simulink model "aircraft_model"  (R2014b)
settings: Solver=ode45  StartTime=0.0  StopTime=10.0  FixedStep=0.001  RelTol=1e-3
values from neighbouring files (symbols this model uses):
  h0 = 1.5    [sim_data.mat]    (also in simulation_framework.m)
  m_p = 0.64    [sim_data.mat]    (also in simulation_framework.m)
  m_phi = 1.21846967915e-05    [sim_data.mat]    (also in simulation_framework.m)
  m_v = 0.25    [sim_data.mat]    (also in simulation_framework.m)
  m_v_air = 0.01    [sim_data.mat]    (also in simulation_framework.m)
  p0 = [2 2]    [sim_data.mat]    (also in simulation_framework.m = [2;2])
  phi_max = 0.523598775598    [sim_data.mat]    (also in simulation_framework.m)
  q = q+q_add    [high_level.m]    (also in start_script.m = 0.005)
  r = d+db/norm(db)*ddr    [lateral_guidance.m]
  seed_p_pdot = [814724 905792 12707 913377 6692 975494]    [sim_data.mat]    (also in simulation_framework.m = [10;2;0.01;2311;132;453287])
  seed_phi = 54689    [sim_data.mat]    (also in simulation_framework.m = 20143)
  seed_v_air = 27849822    [sim_data.mat]    (also in simulation_framework.m = 33)
  Tctrl = 0.1    [sim_data.mat]    (also in simulation_framework.m)
  Ts = 0.1    [sim_data.mat]    (also in simulation_framework.m)
  Ts_p_pdot = 2    [sim_data.mat]    (also in simulation_framework.m)
  Ts_phi = 1    [sim_data.mat]    (also in simulation_framework.m)
  Ts_v_air = 1    [sim_data.mat]    (also in simulation_framework.m)
  VTd = 10    [sim_data.mat]    (also in simulation_framework.m)
  Vw = norm(w)    [findxi.m]    (also in sim_data.mat = 2; simulation_framework.m = 1)
  xi0 = 1.57079632679    [sim_data.mat]    (also in simulation_framework.m = double(findxi(xig0,VTd,w)))
  xiw = atan2(w(2),w(1))    [findxi.m]    (also in sim_data.mat = 4.71238898038; simulation_framework.m = 4.71238898038)
undefined symbols (not defined in the file or in its folder): F, Light, MIL, sigbuilder_block
libraries: aerolibwind2 x2, aerolibtransform2 x1, simulink x1
settings Model: Creator=tstastny  LastModifiedBy=Maverick
settings SolverCC: ZeroCrossAlgorithm=Adaptive
settings OptimizationCC: UseDivisionForNetSlopeComputation=off  SimCompilerOptimization=off
settings DebuggingCC: FrameProcessingCompatibilityMsg=error
settings RTWCC: RTWCompilerOptimization=off

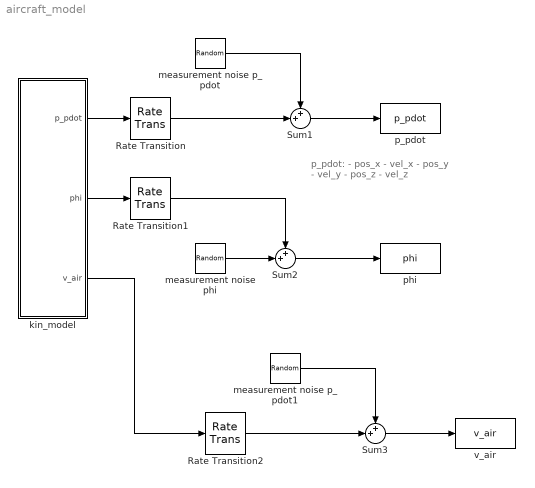
== system aircraft_model ==
  note: p_pdot:  - pos_x
      |               - vel_x
      |               - pos_y
      |               - vel_y
      |               - pos_z
      |               - vel_z
  Rate Transition : RateTransition  Integrity=off  OutPortSampleTime=Ts_p_pdot
  Rate Transition1 : RateTransition  Integrity=off  OutPortSampleTime=Ts_phi
  Rate Transition2 : RateTransition  Integrity=off  OutPortSampleTime=Ts_v_air
  Sum1 : Sum  Inputs=++|  SampleTime=Ts_p_pdot
  Sum2 : Sum  Inputs=++|  SampleTime=Ts_phi
  Sum3 : Sum  Inputs=++|  SampleTime=Ts_v_air
  kin_model : Subsystem
  measurement noise p_pdot : RandomNumber  Variance=[m_p;m_v;m_p;m_v;m_p;m_v]  Seed=seed_p_pdot  SampleTime=Ts_p_pdot
  measurement noise p_pdot1 : RandomNumber  Variance=[m_v_air]  Seed=seed_v_air  SampleTime=Ts_v_air
  measurement noise phi : RandomNumber  Variance=m_phi  Seed=seed_phi  SampleTime=Ts_phi
  p_pdot : ToWorkspace  VariableName=p_pdot  SaveFormat=Structure With Time  SampleTime=-1
  phi : ToWorkspace  VariableName=phi  SaveFormat=Structure With Time  SampleTime=-1
  v_air : ToWorkspace  VariableName=v_air  SaveFormat=Structure With Time  SampleTime=-1
  wires:
  measurement noise p_pdot/1 -> Sum1/1
  measurement noise phi/1 -> Sum2/2
  kin_model/2(phi) -> Rate Transition1/1
  kin_model/1(p_pdot) -> Rate Transition/1
  Rate Transition/1 -> Sum1/2
  Sum1/1 -> p_pdot/1
  Rate Transition1/1 -> Sum2/1
  Sum2/1 -> phi/1
  measurement noise p_pdot1/1 -> Sum3/1
  Rate Transition2/1 -> Sum3/2
  Sum3/1 -> v_air/1
  kin_model/3(v_air) -> Rate Transition2/1

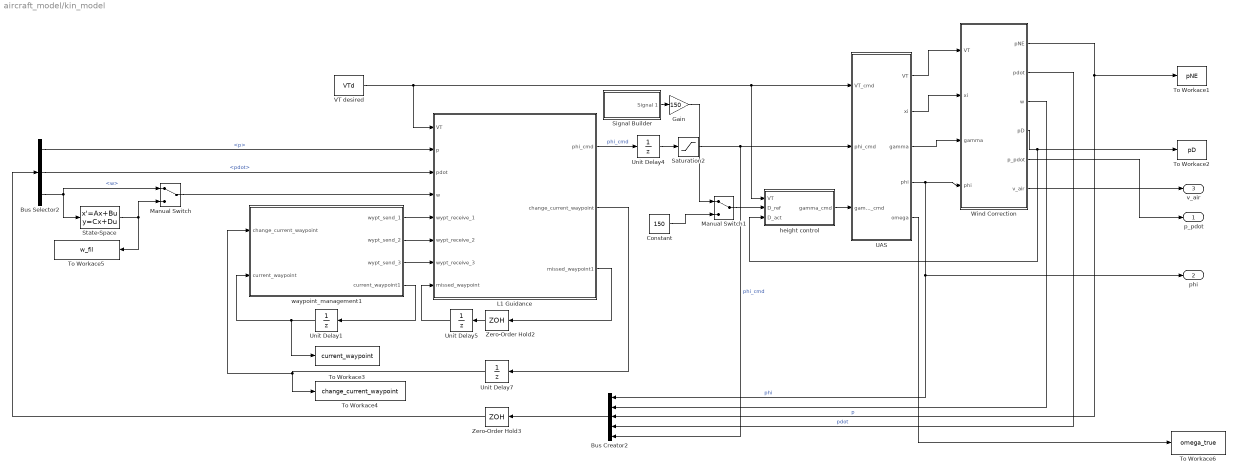
== system aircraft_model/kin_model ==
  Bus Creator2 : BusCreator  Inputs=5
  Bus Selector2 : BusSelector  OutputSignals=p,pdot,w
  Constant : Constant  Value=150  SampleTime=Ts
  Gain : Gain  Gain=150
  L1 Guidance : MATLAB Function  TreatAsAtomicUnit=on  SystemSampleTime=Tctrl
  Manual Switch : ManualSwitch
  Manual Switch1 : ManualSwitch
  Saturation2 : Saturate  UpperLimit=phi_max  LowerLimit=-phi_max
  Signal Builder : Subsystem  Tag=STV Subsys  LoadFcn=sigbuilder_block('load',[0 51 1440 753 ]);  StartFcn=sigbuilder_block('start');  StopFcn=sigbuilder_block('stop');  ClipboardFcn=sigbuilder_block('clipboard');  mask(Sigbuilder block){}
      mask help: Simulink:masks:SigbuilderBlock_MD
      mask init:
      | if ~strcmp(get_param(bdroot(gcbh),'SimulationStatus'),'stopped') tuvar = sigbuilder_block('maskInit'); end
      settings: CopyFcn=sigbuilder_block('copy');  DeleteFcn=sigbuilder_block('delete');  ModelCloseFcn=sigbuilder_block('modelClose');  PreSaveFcn=sigbuilder_block('preSave');  PauseFcn=sigbuilder_block('pause');  ContinueFcn=sigbuilder_block('continue');  NameChangeFcn=sigbuilder_block('namechange');  OpenFcn=sigbuilder_block('open',[437.6 199.2 550.4 400 ]);  CloseFcn=sigbuilder_block('close');
      mask Display: plot(0, 0, 100, 100,[2, 2, 32, 32, 2], [68, 8, 8, 68, 68],[32, 2], [38, 38], [32, 19, 2],[53, 60, 44], [32, 17, 17, 2],[16, 16, 31, 31]);txt = getActiveGroup(gcbh);text(2, 100, txt,'verticalAlignment', 'top');
  State-Space : StateSpace  A=-1*eye(2)  B=1*eye(2)  C=eye(2)  D=zeros(2)  X0=double([Vw*cos(xiw);Vw*sin(xiw)])
  To Workace1 : ToWorkspace  VariableName=pNE  SaveFormat=Structure With Time  SampleTime=Ts
  To Workace2 : ToWorkspace  VariableName=pD  SaveFormat=Structure With Time  SampleTime=Ts
  To Workace3 : ToWorkspace  VariableName=current_waypoint  SaveFormat=Structure With Time  SampleTime=Ts
  To Workace4 : ToWorkspace  VariableName=change_current_waypoint  SaveFormat=Structure With Time  SampleTime=Ts
  To Workace5 : ToWorkspace  VariableName=w_fil  SaveFormat=Structure With Time  SampleTime=Ts
  To Workace6 : ToWorkspace  VariableName=omega_true  SaveFormat=Structure With Time  SampleTime=Ts
  "UAS " : Subsystem
  Unit Delay1 : UnitDelay  InitialCondition=1  SampleTime=0.001
  Unit Delay4 : UnitDelay  SampleTime=0.001
  Unit Delay5 : UnitDelay  SampleTime=0.001
  Unit Delay7 : UnitDelay  SampleTime=0.001
  VT desired : Constant  Value=VTd
  Wind Correction : Subsystem
  Zero-Order Hold2 : ZeroOrderHold  SampleTime=0.001
  Zero-Order Hold3 : ZeroOrderHold  SampleTime=Tctrl
  height control : Subsystem
  waypoint_management1 : MATLAB Function  TreatAsAtomicUnit=on  SystemSampleTime=Tctrl
  p_pdot : Outport
  phi : Outport  Port=2
  v_air : Outport  Port=3
  wires:
  "UAS "/1(VT) -> Wind Correction/1(VT)
  "UAS "/2(xi) -> Wind Correction/2(xi)
  "UAS "/4(phi) -> phi/1, Bus Creator2/1, Wind Correction/4(phi)  "phi"
  Wind Correction/1(pNE) -> Bus Creator2/3, To Workace1/1  "p"
  Wind Correction/2(pdot) -> Bus Creator2/4  "pdot"
  Bus Creator2/1 -> Zero-Order Hold3/1
  Zero-Order Hold3/1 -> Bus Selector2/1
  Bus Selector2/1 -> L1 Guidance/2(p)  "<p>"
  Bus Selector2/2 -> L1 Guidance/3(pdot)  "<pdot>"
  Saturation2/1 -> "UAS "/2(phi_cmd), Bus Creator2/5  "phi_cmd"
  waypoint_management1/4(current_waypoint1) -> Unit Delay1/1
  Unit Delay1/1 -> To Workace3/1, waypoint_management1/2(current_waypoint)
  L1 Guidance/2(change_current_waypoint) -> Unit Delay7/1
  waypoint_management1/3(wypt_send_3) -> L1 Guidance/7(wypt_receive_3)
  waypoint_management1/2(wypt_send_2) -> L1 Guidance/6(wypt_receive_2)
  waypoint_management1/1(wypt_send_1) -> L1 Guidance/5(wypt_receive_1)
  L1 Guidance/3(missed_waypoint1) -> Zero-Order Hold2/1
  Zero-Order Hold2/1 -> Unit Delay5/1
  Wind Correction/3(w) -> Bus Creator2/2
  Bus Selector2/3 -> State-Space/1, Manual Switch/1  "<w>"
  State-Space/1 -> To Workace5/1, Manual Switch/2
  Manual Switch/1 -> L1 Guidance/4(w)
  Unit Delay4/1 -> Saturation2/1
  Unit Delay5/1 -> L1 Guidance/8(missed_waypoint)
  Unit Delay7/1 -> To Workace4/1, waypoint_management1/1(change_current_waypoint)
  L1 Guidance/1(phi_cmd) -> Unit Delay4/1  "phi_cmd"
  Wind Correction/4(pD) -> height control/3(D_act), To Workace2/1
  "UAS "/3(gamma) -> Wind Correction/3(gamma)
  height control/1(gamma_cmd) -> "UAS "/3(gamma_cmd)
  VT desired/1 -> L1 Guidance/1(VT), "UAS "/1(VT_cmd), height control/1(VT)
  Wind Correction/5(p_pdot) -> p_pdot/1
  "UAS "/5(omega) -> To Workace6/1
  Constant/1 -> Manual Switch1/2
  Manual Switch1/1 -> height control/2(D_ref)
  Wind Correction/6(v_air) -> v_air/1
  Gain/1 -> Manual Switch1/1
  Signal Builder/1(Signal 1) -> Gain/1

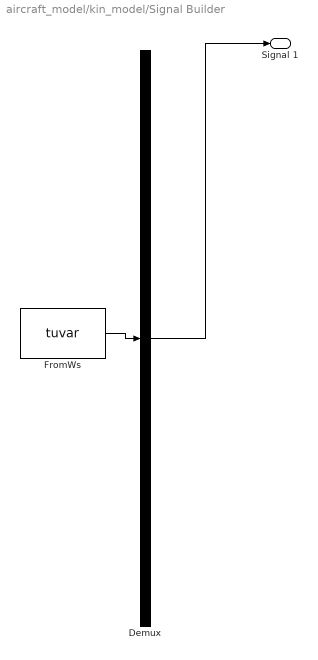
== system aircraft_model/kin_model/Signal Builder ==
  Demux : Demux  Tag=STV Demux  Outputs=1
  FromWs : FromWorkspace  Tag=STV FromWs  VariableName=tuvar  SampleTime=0
      SigBuilderData=|
      | common.afterFinalStr = 'Extrapolate'
      | common.sampleTime = 0
      | dataSet.timeRange = [0 180]
      | dataSet.name = 'Group 1'
      | sbobj.Groups.Name = 'Group 1'
      | sbobj.Groups.Signals.Name = 'Signal 1'
      | sbobj.Groups.Signals.XData = [0 2 10 15 17 20 25 40 60 80 90 100 140 180]
      | sbobj.Groups.Signals.YData = [0 0.008 0.02 0.044 0.052 0.066 0.094 0.192 0.296 0.362 0.362 0.324 0.184 0.048]
      | sbobj.Groups.TimeRange = [0 180]
  Signal 1 : Outport  Tag=STV Outport
  wires:
  Demux/1 -> Signal 1/1
  FromWs/1 -> Demux/1

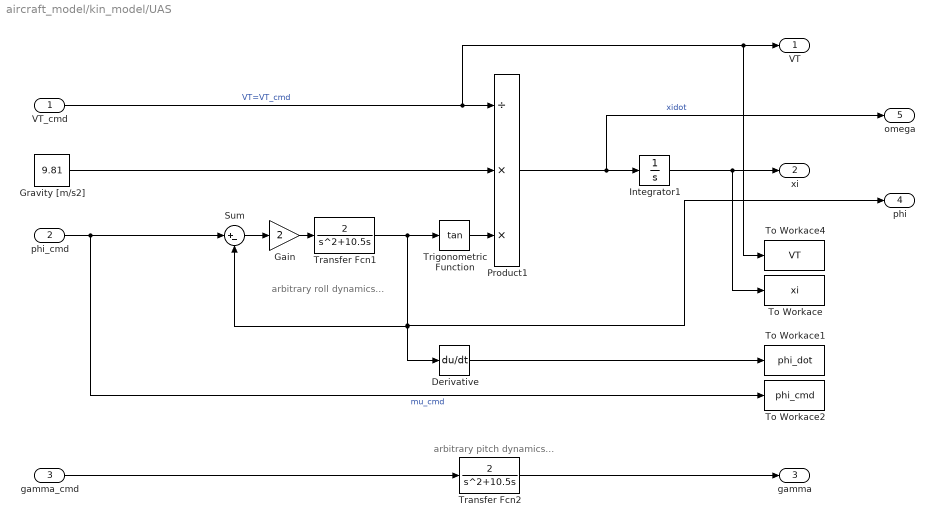
== system aircraft_model/kin_model/UAS  ==
  note: arbitrary roll dynamics...
  note: arbitrary pitch dynamics...
  VT_cmd : Inport
  phi_cmd : Inport  Port=2
  gamma_cmd : Inport  Port=3
  Derivative : Derivative
  Gain : Gain  Gain=2
  Gravity [m/s2] : Constant  Value=9.81
  Integrator1 : Integrator  InitialCondition=xi0
  Product1 : Product  Inputs=/**
  Sum : Sum  Inputs=|+-
  To Workace : ToWorkspace  VariableName=xi  SaveFormat=Structure With Time  SampleTime=Ts
  To Workace1 : ToWorkspace  VariableName=phi_dot  SaveFormat=Structure With Time  SampleTime=Ts
  To Workace2 : ToWorkspace  VariableName=phi_cmd  SaveFormat=Structure With Time  SampleTime=Ts
  To Workace4 : ToWorkspace  VariableName=VT  SaveFormat=Structure With Time  SampleTime=Ts
  Transfer Fcn1 : TransferFcn  Numerator=[2]  Denominator=[1 10.5 0]
  Transfer Fcn2 : TransferFcn  Numerator=[2]  Denominator=[1 10.5 0]
  Trigonometric Function : Trigonometry  Operator=tan
  VT : Outport
  xi : Outport  Port=2
  gamma : Outport  Port=3
  phi : Outport  Port=4
  omega : Outport  Port=5
  wires:
  phi_cmd/1 -> Sum/1, To Workace2/1  "mu_cmd"
  Trigonometric Function/1 -> Product1/3
  Gravity [m/s2]/1 -> Product1/2
  VT_cmd/1 -> To Workace4/1, VT/1, Product1/1  "VT=VT_cmd"
  Product1/1 -> omega/1, Integrator1/1  "xidot"
  Transfer Fcn1/1 -> Derivative/1, Sum/2, phi/1, Trigonometric Function/1
  Derivative/1 -> To Workace1/1
  Gain/1 -> Transfer Fcn1/1
  Sum/1 -> Gain/1
  Integrator1/1 -> To Workace/1, xi/1
  gamma_cmd/1 -> Transfer Fcn2/1
  Transfer Fcn2/1 -> gamma/1

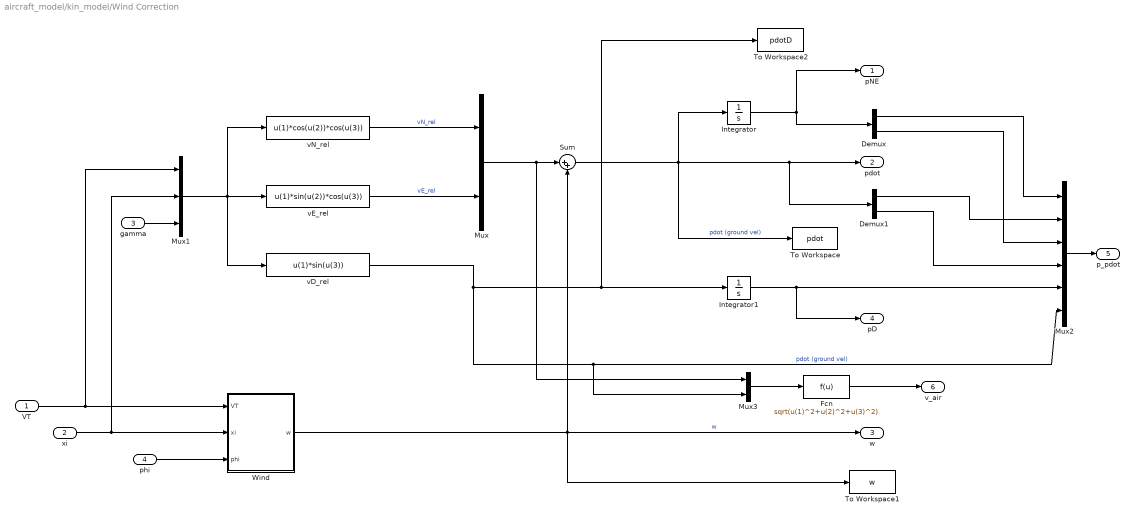
== system aircraft_model/kin_model/Wind Correction ==
  VT : Inport
  xi : Inport  Port=2
  gamma : Inport  Port=3
  phi : Inport  Port=4
  Demux : Demux  Outputs=2
  Demux1 : Demux  Outputs=2
  Fcn : Fcn  Expr=sqrt(u(1)^2+u(2)^2+u(3)^2)
  Integrator : Integrator  InitialCondition=p0
  Integrator1 : Integrator  InitialCondition=h0
  Mux : Mux  Inputs=2
  Mux1 : Mux  Inputs=3
  Mux2 : Mux  Inputs=6
  Mux3 : Mux  Inputs=2
  Sum : Sum  Inputs=|++
  To Workspace : ToWorkspace  VariableName=pdot  SaveFormat=Structure With Time  SampleTime=Ts
  To Workspace1 : ToWorkspace  VariableName=w  SaveFormat=Structure With Time  SampleTime=Ts
  To Workspace2 : ToWorkspace  VariableName=pdotD  SaveFormat=Structure With Time  SampleTime=Ts
  Wind : Subsystem
  vD_rel : Fcn  Expr=u(1)*sin(u(3))  SampleTime=Ts
  vE_rel : Fcn  Expr=u(1)*sin(u(2))*cos(u(3))  SampleTime=Ts
  vN_rel : Fcn  Expr=u(1)*cos(u(2))*cos(u(3))  SampleTime=Ts
  pNE : Outport  PortDimensions=2
  pdot : Outport  Port=2  PortDimensions=2
  w : Outport  Port=3  PortDimensions=2
  pD : Outport  Port=4
  p_pdot : Outport  Port=5
  v_air : Outport  Port=6
  wires:
  VT/1 -> Mux1/1, Wind/1(VT)
  Wind/1(w) -> To Workspace1/1, Sum/2, w/1  "w"
  xi/1 -> Mux1/2, Wind/2(xi)
  phi/1 -> Wind/3(phi)
  Mux/1 -> Mux3/1, Sum/1
  Sum/1 -> Integrator/1, Demux1/1, pdot/1, To Workspace/1  "pdot (ground vel)"
  Integrator/1 -> Demux/1, pNE/1
  gamma/1 -> Mux1/3
  vN_rel/1 -> Mux/1  "vN_rel"
  vE_rel/1 -> Mux/2  "vE_rel"
  Mux1/1 -> vN_rel/1, vD_rel/1, vE_rel/1
  Integrator1/1 -> pD/1, Mux2/5
  vD_rel/1 -> Mux3/2, Mux2/6, To Workspace2/1, Integrator1/1  "pdot (ground vel)"
  Mux2/1 -> p_pdot/1
  Demux/1 -> Mux2/1
  Demux/2 -> Mux2/3
  Demux1/2 -> Mux2/4
  Demux1/1 -> Mux2/2
  Fcn/1 -> v_air/1
  Mux3/1 -> Fcn/1

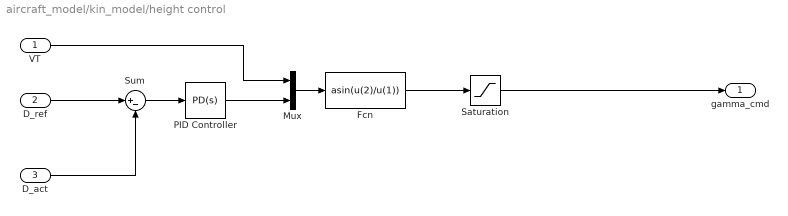
== system aircraft_model/kin_model/height control ==
  VT : Inport
  D_ref : Inport  Port=2
  D_act : Inport  Port=3
  Fcn : Fcn  Expr=asin(u(2)/u(1))  SampleTime=Ts
  Mux : Mux  Inputs=2
  PID Controller : simulink/Continuous/PID Controller  Controller=PD  TimeDomain=Continuous-time  SampleTime=-1  IntegratorMethod=Forward Euler  FilterMethod=Forward Euler  Form=Parallel  P=5  I=1  D=10  N=100  InitialConditionSource=internal  InitialConditionForIntegrator=0  InitialConditionForFilter=0  ExternalReset=none  LimitOutput=off  UpperSaturationLimit=inf  LowerSaturationLimit=-inf  LinearizeAsGain=on  AntiWindupMode=none  Kb=1  TrackingMode=off  Kt=1  PParamMin=[]  PParamMax=[]  IParamMin=[]  IParamMax=[]  DParamMin=[]  DParamMax=[]  NParamMin=[]  NParamMax=[]  KbParamMin=[]  KbParamMax=[]  KtParamMin=[]  KtParamMax=[]  POutMin=[]  POutMax=[]  IOutMin=[]  IOutMax=[]  DOutMin=[]  DOutMax=[]  NOutMin=[]  NOutMax=[]  KbOutMin=[]  KbOutMax=[]  KtOutMin=[]  KtOutMax=[]  IntegratorOutMin=[]  IntegratorOutMax=[]  FilterOutMin=[]  FilterOutMax=[]  SumOutMin=[]  SumOutMax=[]  SumI1OutMin=[]  SumI1OutMax=[]  SumI2OutMin=[]  SumI2OutMax=[]  SumI3OutMin=[]  SumI3OutMax=[]  SumDOutMin=[]  SumDOutMax=[]  SaturationOutMin=[]  SaturationOutMax=[]  IntegratorContinuousStateAttributes=''  IntegratorStateMustResolveToSignalObject=off  IntegratorRTWStateStorageClass=Auto  FilterContinuousStateAttributes=''  FilterStateMustResolveToSignalObject=off  FilterRTWStateStorageClass=Auto  DifferentiatorICPrevScaledInput=0  DifferentiatorOutMin=[]  DifferentiatorOutMax=[]  UseFilter=on
  Saturation : Saturate  UpperLimit=phi_max  LowerLimit=-phi_max
  Sum : Sum  Inputs=|+-
  gamma_cmd : Outport
  wires:
  D_ref/1 -> Sum/1
  Fcn/1 -> Saturation/1
  PID Controller/1 -> Mux/2
  D_act/1 -> Sum/2
  Sum/1 -> PID Controller/1
  VT/1 -> Mux/1
  Mux/1 -> Fcn/1
  Saturation/1 -> gamma_cmd/1

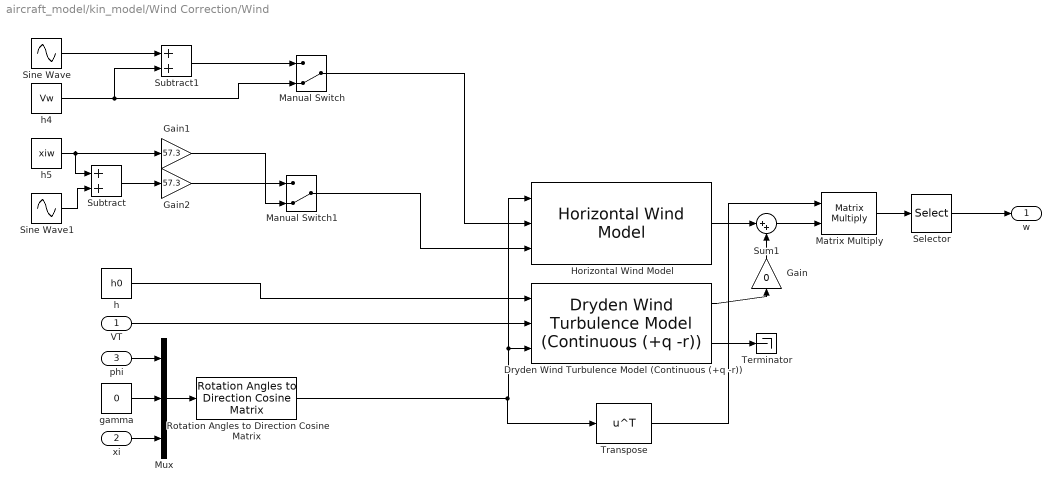
== system aircraft_model/kin_model/Wind Correction/Wind ==
  VT : Inport
  xi : Inport  Port=2
  phi : Inport  Port=3
  Dryden Wind Turbulence Model (Continuous (+q -r)) : aerolibwind2/Dryden Wind Turbulence Model  (Continuous (+q -r))  units=Metric (MKS)  spec=MIL-F-8785C  model=Continuous Dryden (+q -r)  W20=Vw  Wdeg=xiw  TurbProb=10^-2 - Light  L_high=533.4  Wingspan=b_uas  ts=0.01  Seed=[23341 23342 23343 23344]  T_on=on
  Gain : Gain  Gain=0
  Gain1 : Gain  Gain=57.3
  Gain2 : Gain  Gain=57.3
  Horizontal Wind Model : aerolibwind2/Horizontal Wind Model  units=Metric (MKS)  Vw_source=External  Vwind=Vw  W_source=External  Wdeg=xiw
  Manual Switch : ManualSwitch  CurrentSetting=0
  Manual Switch1 : ManualSwitch  CurrentSetting=0
  Matrix Multiply : Product  Multiplication=Matrix(*)
  Mux : Mux  Inputs=3
  Rotation Angles to Direction Cosine Matrix : aerolibtransform2/Rotation Angles to Direction Cosine Matrix  rotationOrder=ZYX
  Selector : Selector  InputPortWidth=3  Indices=[1 2]
  Sine Wave : Sin  Amplitude=3  Bias=-1  Frequency=0.05  SampleTime=0
  Sine Wave1 : Sin  Amplitude=30*pi/180  Frequency=0.1  Phase=35*pi/180  SampleTime=0
  Subtract : Sum
  Subtract1 : Sum
  Sum1 : Sum  Inputs=|++
  Terminator : Terminator
  Transpose : Math  Operator=transpose  SaturateOnIntegerOverflow=on
  gamma : Constant  Value=0
  h : Constant  Value=h0
  h4 : Constant  Value=Vw
  h5 : Constant  Value=xiw
  w : Outport
  wires:
  Dryden Wind Turbulence Model (Continuous (+q -r))/2 -> Terminator/1
  Mux/1 -> Rotation Angles to Direction Cosine Matrix/1
  Rotation Angles to Direction Cosine Matrix/1 -> Transpose/1, Dryden Wind Turbulence Model (Continuous (+q -r))/3, Horizontal Wind Model/1
  h/1 -> Dryden Wind Turbulence Model (Continuous (+q -r))/1
  VT/1 -> Dryden Wind Turbulence Model (Continuous (+q -r))/2
  Horizontal Wind Model/1 -> Sum1/1
  Dryden Wind Turbulence Model (Continuous (+q -r))/1 -> Gain/1
  Transpose/1 -> Matrix Multiply/1
  Sum1/1 -> Matrix Multiply/2
  Selector/1 -> w/1
  Matrix Multiply/1 -> Selector/1
  xi/1 -> Mux/3
  gamma/1 -> Mux/2
  phi/1 -> Mux/1
  Gain/1 -> Sum1/2
  h4/1 -> Manual Switch/2, Subtract1/2
  Sine Wave/1 -> Subtract1/1
  Subtract/1 -> Gain2/1
  h5/1 -> Subtract/1, Gain1/1
  Sine Wave1/1 -> Subtract/2
  Manual Switch1/1 -> Horizontal Wind Model/3
  Manual Switch/1 -> Horizontal Wind Model/2
  Subtract1/1 -> Manual Switch/1
  Gain2/1 -> Manual Switch1/1
  Gain1/1 -> Manual Switch1/2

== matlab function aircraft_model/kin_model/L1 Guidance ==
  data: VT input; p input size=2; pdot input size=2; w input size=2; wypt_receive_1 input Bus: wypt_send_1 size=1; phi_cmd output size=1; wypt_receive_2 input Bus: wypt_send_2 size=1; wypt_receive_3 input Bus: wypt_send_3 size=1; change_current_waypoint output size=1; missed_waypoint input size=1; missed_waypoint1 output size=1
function [phi_cmd,change_current_waypoint,missed_waypoint1] = L1Guidance(VT,p,pdot,w,wypt_receive_1,wypt_receive_2,wypt_receive_3,missed_waypoint)
%#codegen

wypts = [wypt_receive_1,wypt_receive_2,wypt_receive_3];

Rdefault = 70;
sdefault = 1;
change_current_waypoint = 0;
phi_cmd = 0;

% Wind speed estimate greater than airspeed
if norm(w) > 0.99*VT
    
    phi_cmd = 0;%over_airspeed(pdot,w,mumax);
    
elseif ~wypts(1).active && ~wypts(3).active % Only one active waypoint
    
%     [phi_cmd,LAflag] = ...
%         loiter(phi_cmd0,p,pdot,VT,w,g,wypts(2),mumax,loit_opt,LAgain,Lparams);

    phi_cmd = 0;

elseif wypts(2).wtype==1 % Loiter (unlimited, unless MAVLink says otherwise)
    
%     [phi_cmd,LAflag] = ...
%         loiter(phi_cmd0,p,pdot,VT,w,g,wypts(2),mumax,loit_opt,LAgain,Lparams);
    
elseif wypts(2).wtype==0 % Segment tracking
    
    if ~wypts(1).active || missed_waypoint % Inactive wypts 1 or missed wypts 2
        
        if norm(wypts(2).p-p)<wypts(2).param1
            
            if ~wypts(3).active % Terminal loiter
                
%                 [phi_cmd,LAflag] = ...
%                     loiter(phi_cmd0,p,pdot,VT,w,g,wypts(2),mumax,loit_opt,LAgain,Lparams);
                phi_cmd = 0;
                
            else % switch to next wypts pair
                
                a = wypts(2).p;
                b = wypts(3).p;
                phi_cmd = lateral_guidance(p,pdot,a,b);
                
            end
        
            missed_waypoint=0;
            change_current_waypoint=1;
            
        else % L1 guide from p to b
            
            a = p;
            b = wypts(2).p;
            phi_cmd = lateral_guidance(p,pdot,a,b);
        
        end
        
    elseif ~wypts(3).active % Terminal
        
        % check for missed..
        xi_track = atan2(wypts(2).p(2)-wypts(1).p(2),...
            wypts(2).p(2)-wypts(1).p(2));
        HINt = [cos(xi_track) sin(xi_track)];
        if HINt*(p-wypts(1).p) > HINt*(wypts(2).p-wypts(1).p)+wypts(2).param1
            missed_waypoint=1;
        end
        
        if norm(wypts(2).p-p)<wypts(2).param1
        % for now just keep going back to the same... should loiter
            
        	a = p;
            b = wypts(2).p;
            phi_cmd = lateral_guidance(p,pdot,a,b);
            
            change_current_waypoint=1;
            
        elseif missed_waypoint
            
        	a = p;
            b = wypts(2).p;
            phi_cmd = lateral_guidance(p,pdot,a,b);
        
        else
            
            a = wypts(1).p;
            b = wypts(2).p;
            phi_cmd = lateral_guidance(p,pdot,a,b);
        
        end
        
    else
        
        % check for missed..
        xi_track = atan2(wypts(2).p(2)-wypts(1).p(2),...
            wypts(2).p(2)-wypts(1).p(2));
        HINt = [cos(xi_track) sin(xi_track)];
        if HINt*(p-wypts(1).p) > HINt*(wypts(2).p-wypts(1).p)+wypts(2).param1
            missed_waypoint=1;
        end
        
        if norm(wypts(2).p-p)<wypts(2).param1 
            
            a = wypts(2).p;
            b = wypts(3).p;
            phi_cmd = lateral_guidance(p,pdot,a,b);
            
            change_current_waypoint=1;
        
        elseif missed_waypoint
            
            a = p;
            b = wypts(2).p;
            phi_cmd = lateral_guidance(p,pdot,a,b);
            
        else
            
            a = wypts(1).p;
            b = wypts(2).p;
            phi_cmd = lateral_guidance(p,pdot,a,b);
            
        end
             
    end

else % Level aircraft
    
    phi_cmd = 0;
    
end

missed_waypoint1 = missed_waypoint;

== matlab function aircraft_model/kin_model/waypoint_management1 ==
  data: wypts0 parameter size=sizewypts00; change_current_waypoint input size=1; wypt_send_1 output Bus: wypt_send_1 size=1; wypt_send_2 output Bus: wypt_send_2 size=1; wypt_send_3 output Bus: wypt_send_3 size=1; current_waypoint input size=1; current_waypoint1 output size=1
function [wypt_send_1,wypt_send_2,wypt_send_3,current_waypoint1] = ...
    waypoint_management(wypts0,change_current_waypoint,current_waypoint)
%#codegen
% ========================================================================

% This block is intended to mimic Mavlink waypoint switching logic

% ========================================================================

% - - - - - - -
% Waypoint info
% - - - - - - - 

% Empty waypoint
wyptsi = struct('active',0,...
                'wtype',0,...
                'p',zeros(2,1),...
                'param1',30,...
                'param2',0);

% Size of waypoint list
size_waypoint_list = size(wypts0,1);

% - - - - - - - - - - - - - - -
% Determine waypoint send list
% - - - - - - - - - - - - - - -

% Check for change
if change_current_waypoint
    
    % Reached end of list, loop back
    if current_waypoint == size_waypoint_list || size_waypoint_list == 1
        
        current_waypoint = 1;
        
    else
        
        current_waypoint = current_waypoint + 1;
        
    end
    
end

% - - - - - - - - -
% Waypoint send set
% - - - - - - - - - 

if size_waypoint_list == 1
    
    wypt_send_1 = wyptsi;
    wypt_send_2 = wypts0;
    wypt_send_3 = wyptsi;
    
elseif size_waypoint_list == 2
    
    if current_waypoint == size_waypoint_list
        
        wypt_send_1 = wypts0(1);
        wypt_send_2 = wypts0(2);
        wypt_send_3 = wyptsi;
    
    else
        
        wypt_send_1 = wypts0(2);
        wypt_send_2 = wypts0(1);
        wypt_send_3 = wyptsi;
        
    end
    
else
    
    if current_waypoint == size_waypoint_list
        
        wypt_send_1 = wypts0(size_waypoint_list-1);
        wypt_send_2 = wypts0(size_waypoint_list);
        wypt_send_3 = wypts0(1);
        
    elseif current_waypoint == 1
        
        wypt_send_1 = wypts0(size_waypoint_list);
        wypt_send_2 = wypts0(current_waypoint);
        wypt_send_3 = wypts0(current_waypoint+1);
        
    else
        
        wypt_send_1 = wypts0(current_waypoint-1);
        wypt_send_2 = wypts0(current_waypoint);
        wypt_send_3 = wypts0(current_waypoint+1);
        
    end

end

current_waypoint1 = current_waypoint;
